simulink model "modelo_real"  (R2018b)
settings: Solver=ode4  StartTime=0.0  StopTime=t_f  FixedStep=fst  RelTol=1e-3
values from neighbouring files (symbols this model uses):
  b = 0.1210    (= 0.121)    [script_principal.m]
  c_d = r_d/(2*b)    (= 0.120661157025)    [script_principal.m]
  c_e = r_e/(2*b)    (= 0.121074380165)    [script_principal.m]
  delayD = 0.1/fst    (= 100)    [script_principal.m]
  delayE = 0.1/fst    (= 100)    [script_principal.m]
  filter_order = 2    [script_principal.m]
  freq_pos = 200    [script_principal.m]
  freq_vel = 200    [script_principal.m]
  k0 = 10    [script_principal.m]
  k_enc = 2*pi/fpr    (= 0.157079632679)    [script_principal.m]
  KaD_v = var_KaD*0.4713    (= 0.4713)    [script_principal.m]
  KaE_v = var_KaE*0.5046    (= 0.5046)    [script_principal.m]
  L = 0.1    [script_principal.m]
  svzD = 0    [script_principal.m]
  svzE = 0    [script_principal.m]
  T = 3    [script_principal.m]
  VaD_max = 14    [script_principal.m]
  VaD_min = 2    [script_principal.m]
  VaE_max = 14    [script_principal.m]
  VaE_min = 2    [script_principal.m]
  x0_1 = 0    [script_principal.m]
  x0_2 = 0    [script_principal.m]
  x0_3 = 0    [script_principal.m]
undefined symbols (not defined in the file or in its folder): a, dur_c, t_f, t_i, t_i_1, t_i_2, t_i_3, t_i_c, time_c, v, w, wx, wy
libraries: simulink x39, embdlinuxlib x7, cstblocks x4, dspmtrx3 x2, raspberrypilib x1
settings Model: SimulationMode=external  ExtModeTrigDuration=2  Creator=nenem  LastModifiedBy=nenem
settings SolverCC: PositivePriorityOrder=on
settings OptimizationCC: EnhancedBackFolding=on  PassReuseOutputArgsAs=Individual arguments  MaxStackSize=64  OptimizeBlockOrder=speed  DifferentSizesBufferReuse=on  OptimizationCustomize=off
settings DebuggingCC: ParameterTunabilityLossMsg=error
settings HardwareCC: ProdBitPerPointer=32  ProdBitPerSizeT=32  ProdBitPerPtrDiffT=32  ProdLargestAtomicInteger=Long  ProdLargestAtomicFloat=Double  ProdWordSize=32  ProdHWDeviceType=ARM Compatible->ARM Cortex
settings SFSimCC: MATLABDynamicMemAlloc=off
settings RTWCC: SystemTargetFile=ert.tlc  HardwareBoard=Raspberry Pi  TLCOptions="-aInlineSetEventsForThisBaseRateFcn=TLC_FALSE -aSuppressMultiTaskScheduler=TLC_FALSE  -aRateBasedStepFcn=0"  TemplateMakefile=ert_default_tmf  GenerateReport=on  Toolchain=GNU GCC Raspberry Pi  BuildConfiguration=Faster Runs  IncludeHyperlinkInReport=on  LaunchReport=on  GenerateTraceInfo=on  GenerateTraceReport=on  GenerateTraceReportSl=on  GenerateTraceReportSf=on  GenerateTraceReportEml=on
settings CodeAppCC: ForceParamTrailComments=on  IgnoreCustomStorageClasses=off  OperatorAnnotations=on  SimulinkDataObjDesc=on  SFDataObjDesc=on  InsertBlockDesc=on
settings ERTTargetCC: SupportContinuousTime=on  SupportVariableSizeSignals=on

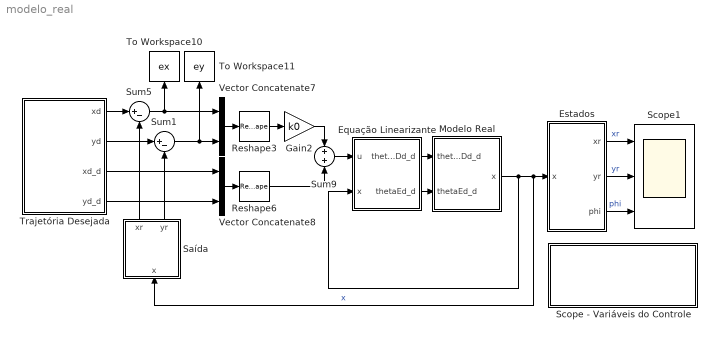
== system modelo_real ==
  Equação Linearizante : Subsystem
  Estados : Subsystem
  Gain2 : Gain  Gain=k0
  Modelo Real : Subsystem
  Reshape3 : Reshape  OutputDimensionality=Customize  OutputDimensions=[2,1]
  Reshape6 : Reshape  OutputDimensionality=Customize  OutputDimensions=[2,1]
  Saída : Subsystem
  Scope - Variáveis do Controle : Subsystem
  Scope1 : Scope  NumInputPorts=3
  Sum1 : Sum  Inputs=|+-
  Sum5 : Sum  Inputs=|+-
  Sum9 : Sum  Inputs=+|+
  To Workspace10 : ToWorkspace  VariableName=ex  SaveFormat=Structure With Time  SampleTime=-1
      settings: Save2DSignal=2-D array (concatenate along first dimension)
  To Workspace11 : ToWorkspace  VariableName=ey  SaveFormat=Structure With Time  SampleTime=-1
      settings: Save2DSignal=2-D array (concatenate along first dimension)
  Trajetória Desejada : Subsystem
  Vector Concatenate7 : Concatenate
  Vector Concatenate8 : Concatenate
  wires:
  Trajetória Desejada/1(xd) -> Sum5/1
  Sum1/1 -> To Workspace11/1, Vector Concatenate7/2
  Gain2/1 -> Sum9/1
  Reshape6/1 -> Sum9/2
  Estados/2(yr) -> Scope1/2  "yr"
  Sum5/1 -> To Workspace10/1, Vector Concatenate7/1
  Trajetória Desejada/4(yd_d) -> Vector Concatenate8/2
  Trajetória Desejada/3(xd_d) -> Vector Concatenate8/1
  Trajetória Desejada/2(yd) -> Sum1/1
  Vector Concatenate7/1 -> Reshape3/1
  Estados/1(xr) -> Scope1/1  "xr"
  Reshape3/1 -> Gain2/1
  Sum9/1 -> Equação Linearizante/1(u)
  Saída/2(yr) -> Sum1/2
  Vector Concatenate8/1 -> Reshape6/1
  Modelo Real/1(x) -> Equação Linearizante/2(x), Saída/1(x), Estados/1(x)  "x"
  Saída/1(xr) -> Sum5/2
  Estados/3(phi) -> Scope1/3  "phi"
  Equação Linearizante/2(thetaEd_d) -> Modelo Real/2(thetaEd_d)
  Equação Linearizante/1(thetaDd_d) -> Modelo Real/1(thetaDd_d)

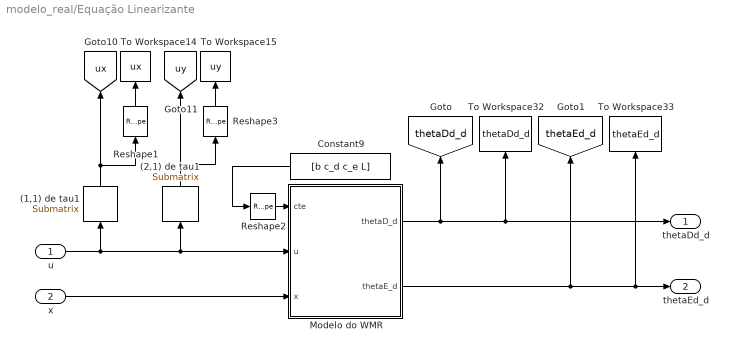
== system modelo_real/Equação Linearizante ==
  u : Inport
  x : Inport  Port=2
  (1,1) de tau1 : dspmtrx3/Submatrix  RowSpan=One row  RowStartMode=Index  RowStartIndex=1  RowEndMode=Last  RowEndIndex=1  ColSpan=One column  ColStartMode=Index  ColStartIndex=1  ColEndMode=Last  ColEndIndex=1
  (2,1) de tau1 : dspmtrx3/Submatrix  RowSpan=One row  RowStartMode=Index  RowStartIndex=2  RowEndMode=Last  RowEndIndex=1  ColSpan=One column  ColStartMode=Index  ColStartIndex=1  ColEndMode=Last  ColEndIndex=1
  Constant9 : Constant  Value=[b c_d c_e L]
  Modelo do WMR : MATLAB Function  TreatAsAtomicUnit=on
  Reshape1 : Reshape
  Reshape2 : Reshape  OutputDimensionality=Customize  OutputDimensions=[1,4]
  Reshape3 : Reshape
  To Workspace14 : ToWorkspace  VariableName=ux  SaveFormat=Structure With Time  SampleTime=-1
      settings: Save2DSignal=2-D array (concatenate along first dimension)
  To Workspace15 : ToWorkspace  VariableName=uy  SaveFormat=Structure With Time  SampleTime=-1
      settings: Save2DSignal=2-D array (concatenate along first dimension)
  To Workspace32 : ToWorkspace  VariableName=thetaDd_d  SaveFormat=Structure With Time  SampleTime=-1
      settings: Save2DSignal=2-D array (concatenate along first dimension)
  To Workspace33 : ToWorkspace  VariableName=thetaEd_d  SaveFormat=Structure With Time  SampleTime=-1
      settings: Save2DSignal=2-D array (concatenate along first dimension)
  thetaDd_d : Outport
  thetaEd_d : Outport  Port=2
  tag scope: thetaDd_d=global, thetaEd_d=global, ux=global, uy=global
  wires:
  x/1 -> Modelo do WMR/3(x)
  Reshape2/1 -> Modelo do WMR/1(cte)
  Constant9/1 -> Reshape2/1
  u/1 -> (1,1) de tau1/1, (2,1) de tau1/1, Modelo do WMR/2(u)
  (2,1) de tau1/1 -> Reshape3/1, [uy]
  (1,1) de tau1/1 -> Reshape1/1, [ux]
  Modelo do WMR/1(thetaD_d) -> [thetaDd_d], To Workspace32/1, thetaDd_d/1
  Modelo do WMR/2(thetaE_d) -> thetaEd_d/1, To Workspace33/1, [thetaEd_d]
  Reshape1/1 -> To Workspace14/1
  Reshape3/1 -> To Workspace15/1

== system modelo_real/Estados ==
  x : Inport
  Estados : MATLAB Function  TreatAsAtomicUnit=on
  To Workspace2 : ToWorkspace  VariableName=phi  SaveFormat=Structure With Time  SampleTime=-1
      settings: Save2DSignal=2-D array (concatenate along first dimension)
  To Workspace3 : ToWorkspace  VariableName=xr  SaveFormat=Structure With Time  SampleTime=-1
      settings: Save2DSignal=2-D array (concatenate along first dimension)
  To Workspace4 : ToWorkspace  VariableName=yr  SaveFormat=Structure With Time  SampleTime=-1
      settings: Save2DSignal=2-D array (concatenate along first dimension)
  xr : Outport
  yr : Outport  Port=2
  phi : Outport  Port=3
  tag scope: phi=global, xr=global, yr=global
  wires:
  x/1 -> Estados/1(x)
  Estados/1(xr) -> xr/1, To Workspace3/1, [xr]
  Estados/2(yr) -> [yr], yr/1, To Workspace4/1
  Estados/3(phi) -> phi/1, To Workspace2/1, [phi]

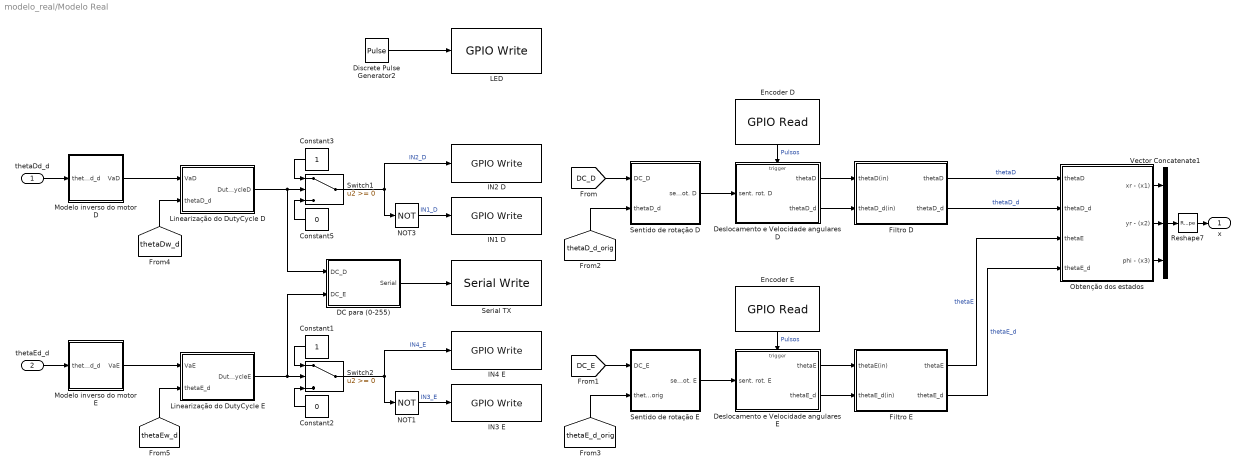
== system modelo_real/Modelo Real ==
  thetaDd_d : Inport
  thetaEd_d : Inport  Port=2
  Constant1 : Constant
  Constant2 : Constant  Value=0
  Constant3 : Constant
  Constant5 : Constant  Value=0
  DC para (0-255) : Subsystem
  Deslocamento e Velocidade angulares D : Subsystem  TreatAsAtomicUnit=on
  Deslocamento e Velocidade angulares E : Subsystem  TreatAsAtomicUnit=on
  Discrete Pulse Generator2 : DiscretePulseGenerator  SampleTime=0.25
  Encoder D : embdlinuxlib/GPIO Read  board=Pi 3 Model B  gpio=26  internalResistor=Off  sampleTime=0.001  direction=Input  blockPlatform=Raspberry Pi
      settings: SourceProductName=Simulink Support Package for Raspberry Pi Hardware  SourceProductBaseCode=RASPPI
  Encoder E : embdlinuxlib/GPIO Read  board=Pi 3 Model B  gpio=5  internalResistor=Off  sampleTime=0.001  direction=Input  blockPlatform=Raspberry Pi
      settings: SourceProductName=Simulink Support Package for Raspberry Pi Hardware  SourceProductBaseCode=RASPPI
  Filtro D : Subsystem
  Filtro E : Subsystem
  IN1 D : embdlinuxlib/GPIO Write  board=Pi 3 Model B  gpio=16  direction=Output  blockPlatform=Raspberry Pi
      settings: SourceProductName=Simulink Support Package for Raspberry Pi Hardware  SourceProductBaseCode=RASPPI
  IN2 D : embdlinuxlib/GPIO Write  board=Pi 3 Model B  gpio=20  direction=Output  blockPlatform=Raspberry Pi
      settings: SourceProductName=Simulink Support Package for Raspberry Pi Hardware  SourceProductBaseCode=RASPPI
  IN3 E : embdlinuxlib/GPIO Write  board=Pi 3 Model B  gpio=19  direction=Output  blockPlatform=Raspberry Pi
      settings: SourceProductName=Simulink Support Package for Raspberry Pi Hardware  SourceProductBaseCode=RASPPI
  IN4 E : embdlinuxlib/GPIO Write  board=Pi 3 Model B  gpio=6  direction=Output  blockPlatform=Raspberry Pi
      settings: SourceProductName=Simulink Support Package for Raspberry Pi Hardware  SourceProductBaseCode=RASPPI
  LED : embdlinuxlib/GPIO Write  board=Pi 3 Model B  gpio=21  direction=Output  blockPlatform=Raspberry Pi
      settings: SourceProductName=Simulink Support Package for Raspberry Pi Hardware  SourceProductBaseCode=RASPPI
  Linearização do DutyCycle D : Subsystem
  Linearização do DutyCycle E : Subsystem
  Modelo inverso do motor D : Subsystem
  Modelo inverso do motor E : Subsystem
  NOT1 : Logic  Operator=NOT  IconShape=distinctive  AllPortsSameDT=off  OutDataTypeStr=boolean
  NOT3 : Logic  Operator=NOT  IconShape=distinctive  AllPortsSameDT=off  OutDataTypeStr=boolean
  Obtenção dos estados : Subsystem
  Reshape7 : Reshape  OutputDimensionality=Customize  OutputDimensions=[3,1]
  Sentido de rotação D : Subsystem
  Sentido de rotação E : Subsystem
  Serial TX : raspberrypilib/Serial Write  board=Pi 3 Model B  SCIModule_=/dev/ttyS0  Baudrate_=230400  Parity=None  StopBits_=1  HardwareFlowControl=None  ByteOrder=LittleEndian  OutputStatus=off  blockPlatform=RaspberryPi
      settings: SourceProductName=Simulink Support Package for Raspberry Pi Hardware  SourceProductBaseCode=RASPPI
  Switch1 : Switch
  Switch2 : Switch
  Vector Concatenate1 : Concatenate  NumInputs=3
  x : Outport
  wires:
  Filtro D/1(thetaD) -> Obtenção dos estados/1(thetaD)  "thetaD"
  Switch1/1 -> IN2 D/1, NOT3/1  "IN2_D"
  Filtro E/1(thetaE) -> Obtenção dos estados/3(thetaE)  "thetaE"
  Sentido de rotação D/1(sent. rot. D) -> Deslocamento e Velocidade angulares D/1(sent. rot. D)
  Sentido de rotação E/1(sent. rot. E) -> Deslocamento e Velocidade angulares E/1(sent. rot. E)
  Encoder E/1 -> Deslocamento e Velocidade angulares E/Trigger  "Pulsos"
  NOT3/1 -> IN1 D/1  "IN1_D"
  Switch2/1 -> IN4 E/1, NOT1/1  "IN4_E"
  [DC_D] -> Sentido de rotação D/1(DC_D)
  Encoder D/1 -> Deslocamento e Velocidade angulares D/Trigger  "Pulsos"
  Discrete Pulse Generator2/1 -> LED/1
  Vector Concatenate1/1 -> Reshape7/1
  Filtro D/2(thetaD_d) -> Obtenção dos estados/2(thetaD_d)  "thetaD_d"
  Filtro E/2(thetaE_d) -> Obtenção dos estados/4(thetaE_d)  "thetaE_d"
  [DC_E] -> Sentido de rotação E/1(DC_E)
  thetaDd_d/1 -> Modelo inverso do motor D/1(thetaDd_d)
  Modelo inverso do motor D/1(VaD) -> Linearização do DutyCycle D/1(VaD)
  Linearização do DutyCycle D/1(DutyCycleD) -> DC para (0-255)/1(DC_D), Switch1/2
  thetaEd_d/1 -> Modelo inverso do motor E/1(thetaEd_d)
  Modelo inverso do motor E/1(VaE) -> Linearização do DutyCycle E/1(VaE)
  Linearização do DutyCycle E/1(DutyCycleE) -> DC para (0-255)/2(DC_E), Switch2/2
  DC para (0-255)/1(Serial) -> Serial TX/1
  Constant3/1 -> Switch1/1
  Constant5/1 -> Switch1/3
  Constant1/1 -> Switch2/1
  Constant2/1 -> Switch2/3
  Deslocamento e Velocidade angulares D/1(thetaD) -> Filtro D/1(thetaD(in))
  Deslocamento e Velocidade angulares D/2(thetaD_d) -> Filtro D/2(thetaD_d(in))
  Deslocamento e Velocidade angulares E/1(thetaE) -> Filtro E/1(thetaE(in))
  Deslocamento e Velocidade angulares E/2(thetaE_d) -> Filtro E/2(thetaE_d(in))
  Reshape7/1 -> x/1
  Obtenção dos estados/1(xr - (x1)) -> Vector Concatenate1/1
  Obtenção dos estados/2(yr - (x2)) -> Vector Concatenate1/2
  Obtenção dos estados/3(phi - (x3)) -> Vector Concatenate1/3
  NOT1/1 -> IN3 E/1  "IN3_E"
  [thetaD_d_orig] -> Sentido de rotação D/2(thetaD_d)
  [thetaE_d_orig] -> Sentido de rotação E/2(thetaE_d_orig)
  [thetaDw_d] -> Linearização do DutyCycle D/2(thetaD_d)
  [thetaEw_d] -> Linearização do DutyCycle E/2(thetaE_d)

== system modelo_real/Saída ==
  x : Inport
  Reshape1 : Reshape  OutputDimensionality=Customize  OutputDimensions=[3,1]
  Saídas : MATLAB Function  TreatAsAtomicUnit=on
  xr : Outport
  yr : Outport  Port=2
  wires:
  x/1 -> Reshape1/1
  Saídas/1(xr) -> xr/1
  Saídas/2(yr) -> yr/1
  Reshape1/1 -> Saídas/1(x)

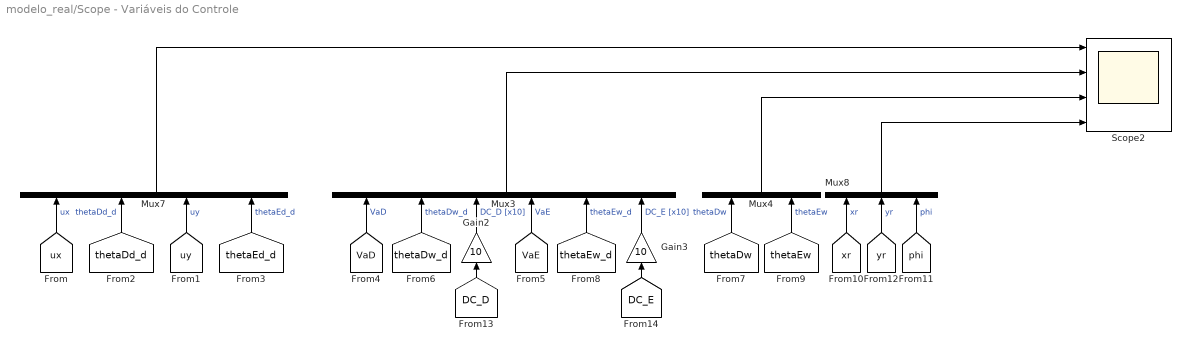
== system modelo_real/Scope - Variáveis do Controle ==
  Gain2 : Gain  Gain=10
  Gain3 : Gain  Gain=10
  Mux3 : Mux  Inputs=6
  Mux4 : Mux  Inputs=2
  Mux7 : Mux
  Mux8 : Mux  Inputs=3
  Scope2 : Scope  NumInputPorts=4
  wires:
  [ux] -> Mux7/1  "ux"
  [thetaDw] -> Mux4/1  "thetaDw"
  [thetaEw_d] -> Mux3/5  "thetaEw_d"
  [phi] -> Mux8/3  "phi"
  [thetaDw_d] -> Mux3/2  "thetaDw_d"
  Mux4/1 -> Scope2/3
  [xr] -> Mux8/1  "xr"
  [thetaEw] -> Mux4/2  "thetaEw"
  Mux7/1 -> Scope2/1
  [yr] -> Mux8/2  "yr"
  [uy] -> Mux7/3  "uy"
  [thetaEd_d] -> Mux7/4  "thetaEd_d"
  Mux8/1 -> Scope2/4
  [VaE] -> Mux3/4  "VaE"
  [VaD] -> Mux3/1  "VaD"
  [thetaDd_d] -> Mux7/2  "thetaDd_d"
  Mux3/1 -> Scope2/2
  [DC_D] -> Gain2/1
  [DC_E] -> Gain3/1
  Gain2/1 -> Mux3/3  "DC_D [x10]"
  Gain3/1 -> Mux3/6  "DC_E [x10]"

== system modelo_real/Trajetória Desejada ==
  Hypot : Math  Operator=hypot  OutputSignalType=real  SaturateOnIntegerOverflow=on
  Integrator : Integrator
  Integrator1 : Integrator
  To Workspace : ToWorkspace  VariableName=vd  SaveFormat=Structure With Time  SampleTime=-1
      settings: Save2DSignal=2-D array (concatenate along first dimension)
  To Workspace1 : ToWorkspace  VariableName=xd  SaveFormat=Structure With Time  SampleTime=-1
      settings: Save2DSignal=2-D array (concatenate along first dimension)
  To Workspace2 : ToWorkspace  VariableName=yd  SaveFormat=Structure With Time  SampleTime=-1
      settings: Save2DSignal=2-D array (concatenate along first dimension)
  To Workspace5 : ToWorkspace  VariableName=xd_d  SaveFormat=Structure With Time  SampleTime=-1
      settings: Save2DSignal=2-D array (concatenate along first dimension)
  To Workspace6 : ToWorkspace  VariableName=yd_d  SaveFormat=Structure With Time  SampleTime=-1
      settings: Save2DSignal=2-D array (concatenate along first dimension)
  Velocidade da trajetória : Subsystem
  xd : Outport
  yd : Outport  Port=2
  xd_d : Outport  Port=3
  yd_d : Outport  Port=4
  wires:
  Integrator/1 -> xd/1, To Workspace1/1  "xd"
  Integrator1/1 -> yd/1, To Workspace2/1  "yd"
  Hypot/1 -> To Workspace/1
  Velocidade da trajetória/1(xd_d) -> Integrator/1, xd_d/1, To Workspace5/1, Hypot/1  "xd_d"
  Velocidade da trajetória/2(yd_d) -> Integrator1/1, yd_d/1, To Workspace6/1, Hypot/2  "yd_d"

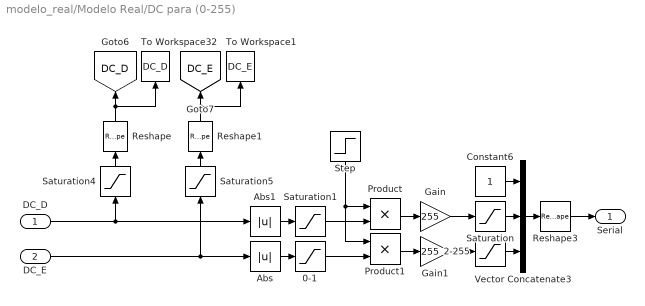
== system modelo_real/Modelo Real/DC para (0-255) ==
  DC_D : Inport
  DC_E : Inport  Port=2
  0-1 : Saturate  UpperLimit=1  LowerLimit=0
  2-255 : Saturate  UpperLimit=255  LowerLimit=2
  Abs : Abs
  Abs1 : Abs
  Constant6 : Constant  OutDataTypeStr=uint8
  Gain : Gain  Gain=255  OutDataTypeStr=uint8
  Gain1 : Gain  Gain=255  OutDataTypeStr=uint8
  Product : Product
  Product1 : Product
  Reshape : Reshape
  Reshape1 : Reshape
  Reshape3 : Reshape  OutputDimensionality=Column vector (2-D)  OutputDimensions=[3,1]
  Saturation : Saturate  UpperLimit=255  LowerLimit=2
  Saturation1 : Saturate  UpperLimit=1  LowerLimit=0
  Saturation4 : Saturate  UpperLimit=1  LowerLimit=-1
  Saturation5 : Saturate  UpperLimit=1  LowerLimit=-1
  Step : Step  Time=t_f-0.01  Before=1  After=0  SampleTime=0
  To Workspace1 : ToWorkspace  VariableName=DC_E  SaveFormat=Structure With Time  SampleTime=-1
      settings: Save2DSignal=2-D array (concatenate along first dimension)
  To Workspace32 : ToWorkspace  VariableName=DC_D  SaveFormat=Structure With Time  SampleTime=-1
      settings: Save2DSignal=2-D array (concatenate along first dimension)
  Vector Concatenate3 : Concatenate  NumInputs=3  ConcatenateDimension=5
  Serial : Outport
  tag scope: DC_D=global, DC_E=global
  wires:
  DC_E/1 -> Abs/1, Saturation5/1
  Saturation/1 -> Vector Concatenate3/2
  DC_D/1 -> Abs1/1, Saturation4/1
  Constant6/1 -> Vector Concatenate3/1
  2-255/1 -> Vector Concatenate3/3
  Vector Concatenate3/1 -> Reshape3/1
  Reshape3/1 -> Serial/1
  Saturation4/1 -> Reshape/1
  Saturation5/1 -> Reshape1/1
  Abs/1 -> 0-1/1
  Abs1/1 -> Saturation1/1
  0-1/1 -> Product1/2
  Saturation1/1 -> Product/2
  Reshape/1 -> To Workspace32/1, [DC_D]
  Reshape1/1 -> To Workspace1/1, [DC_E]
  Gain/1 -> Saturation/1
  Gain1/1 -> 2-255/1
  Step/1 -> Product1/1, Product/1
  Product/1 -> Gain/1
  Product1/1 -> Gain1/1

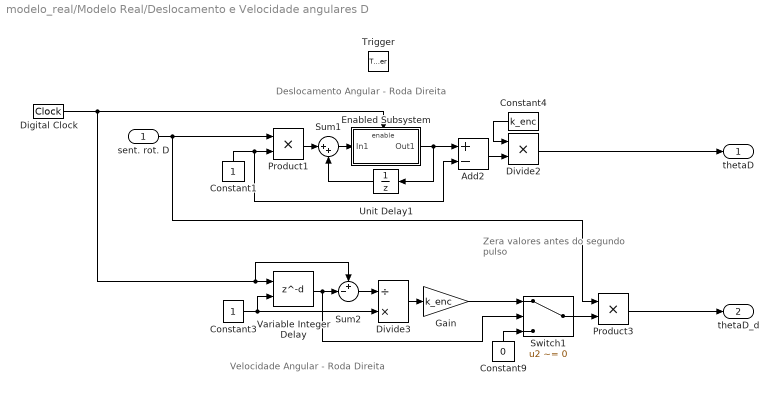
== system modelo_real/Modelo Real/Deslocamento e Velocidade angulares D ==
  note: Deslocamento Angular - Roda Direita
  note: Velocidade Angular - Roda Direita
  note: Zera valores antes
      | do segundo pulso
  sent. rot. D : Inport  LatchByDelayingOutsideSignal=on
  Trigger : TriggerPort  VariantControl=Variant
  Add2 : Sum  Inputs=+-
  Constant1 : Constant  OutDataTypeStr=double
  Constant3 : Constant  OutDataTypeStr=double
  Constant4 : Constant  Value=k_enc  OutDataTypeStr=double
  Constant9 : Constant  Value=0  OutDataTypeStr=double
  Digital Clock : DigitalClock  SampleTime=-1
  Divide2 : Product  Inputs=**  RndMeth=Nearest
  Divide3 : Product  Inputs=/*  RndMeth=Nearest
  Enabled Subsystem : Subsystem  TreatAsAtomicUnit=on
  Gain : Gain  Gain=k_enc
  Product1 : Product
  Product3 : Product
  Sum1 : Sum  Inputs=|++
  Sum2 : Sum  Inputs=+-|
  Switch1 : Switch  Criteria=u2 ~= 0
  Unit Delay1 : UnitDelay  SampleTime=-1
  Variable Integer Delay : Delay  DelayLengthSource=Input port
      settings: InputPortMap=u0,p1
  thetaD : Outport
  thetaD_d : Outport  Port=2
  wires:
  Constant1/1 -> Add2/2, Product1/2
  Enabled Subsystem/1(Out1) -> Add2/1, Unit Delay1/1
  Sum1/1 -> Enabled Subsystem/1(In1)
  Add2/1 -> Divide2/2
  Unit Delay1/1 -> Sum1/2
  Constant4/1 -> Divide2/1
  Product1/1 -> Sum1/1
  Divide3/1 -> Gain/1
  Digital Clock/1 -> Enabled Subsystem/Enable, Variable Integer Delay/1, Sum2/1
  Constant9/1 -> Switch1/3
  Variable Integer Delay/1 -> Sum2/2, Switch1/2
  Switch1/1 -> Product3/2
  Sum2/1 -> Divide3/1
  sent. rot. D/1 -> Product1/1, Product3/1
  Gain/1 -> Switch1/1
  Product3/1 -> thetaD_d/1
  Constant3/1 -> Divide3/2, Variable Integer Delay/2
  Divide2/1 -> thetaD/1

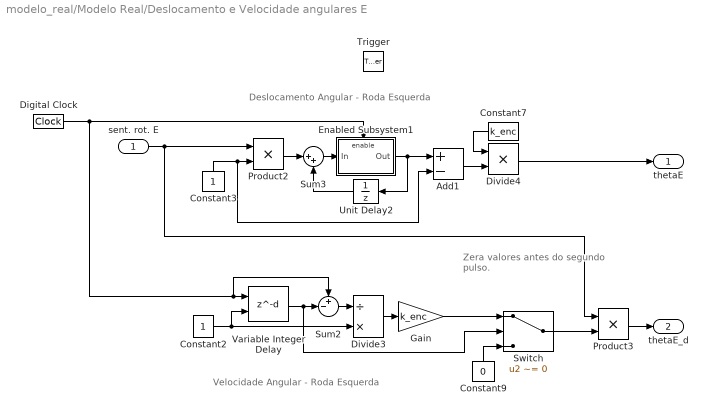
== system modelo_real/Modelo Real/Deslocamento e Velocidade angulares E ==
  note: Deslocamento Angular - Roda Esquerda
  note: Zera valores antes
      | do segundo pulso.
  note: Velocidade Angular - Roda Esquerda
  sent. rot. E : Inport  LatchByDelayingOutsideSignal=on
  Trigger : TriggerPort  VariantControl=Variant
  Add1 : Sum  Inputs=+-
  Constant2 : Constant  OutDataTypeStr=double
  Constant3 : Constant  OutDataTypeStr=double
  Constant7 : Constant  Value=k_enc  OutDataTypeStr=double
  Constant9 : Constant  Value=0  OutDataTypeStr=double
  Digital Clock : DigitalClock  SampleTime=-1
  Divide3 : Product  Inputs=/*  RndMeth=Nearest
  Divide4 : Product  Inputs=**  RndMeth=Nearest
  Enabled Subsystem1 : Subsystem  TreatAsAtomicUnit=on
  Gain : Gain  Gain=k_enc
  Product2 : Product
  Product3 : Product
  Sum2 : Sum  Inputs=+-|
  Sum3 : Sum  Inputs=|++
  Switch : Switch  Criteria=u2 ~= 0
  Unit Delay2 : UnitDelay  SampleTime=-1
  Variable Integer Delay : Delay  DelayLengthSource=Input port
      settings: InputPortMap=u0,p1
  thetaE : Outport
  thetaE_d : Outport  Port=2
  wires:
  Constant2/1 -> Divide3/2, Variable Integer Delay/2
  Product2/1 -> Sum3/1
  Digital Clock/1 -> Enabled Subsystem1/Enable, Variable Integer Delay/1, Sum2/1
  Sum2/1 -> Divide3/1
  Add1/1 -> Divide4/2
  Constant7/1 -> Divide4/1
  Sum3/1 -> Enabled Subsystem1/1(In)
  Constant9/1 -> Switch/3
  Enabled Subsystem1/1(Out) -> Add1/1, Unit Delay2/1
  Switch/1 -> Product3/2
  Unit Delay2/1 -> Sum3/2
  Variable Integer Delay/1 -> Switch/2, Sum2/2
  Constant3/1 -> Add1/2, Product2/2
  sent. rot. E/1 -> Product3/1, Product2/1
  Divide3/1 -> Gain/1
  Gain/1 -> Switch/1
  Product3/1 -> thetaE_d/1
  Divide4/1 -> thetaE/1

== system modelo_real/Modelo Real/Filtro D ==
  thetaD(in) : Inport
  thetaD_d(in) : Inport  Port=2
  Constant : Constant  Value=freq_vel
  Constant1 : Constant  Value=freq_pos
  Constant6 : Constant  Value=0
  Manual Switch : ManualSwitch  CurrentSetting=0
  Média : MATLAB Function  TreatAsAtomicUnit=on
  Sum : Sum  Inputs=+-|
  Switch3 : Switch  Criteria=u2 ~= 0
  Tapped Delay : simulink/Discrete/Tapped Delay  vinit=0.0  samptime=fst  NumDelays=delayD  DelayOrder=Oldest  includeCurrent=off
  To Workspace1 : ToWorkspace  VariableName=thetaD_orig  SaveFormat=Structure With Time  SampleTime=-1
      settings: Save2DSignal=2-D array (concatenate along first dimension)
  To Workspace32 : ToWorkspace  VariableName=thetaD_d_orig  SaveFormat=Structure With Time  SampleTime=-1
      settings: Save2DSignal=2-D array (concatenate along first dimension)
  Unit Delay2 : UnitDelay  SampleTime=-1
  Varying Lowpass Filter : cstblocks/Linear Parameter Varying/Varying Lowpass Filter  N=filter_order
      settings: SourceProductName=Control System Toolbox
  Varying Lowpass Filter1 : cstblocks/Linear Parameter Varying/Varying Lowpass Filter  N=filter_order
      settings: SourceProductName=Control System Toolbox
  thetaD : Outport
  thetaD_d : Outport  Port=2
  tag scope: thetaD_d_orig=global
  wires:
  Constant6/1 -> Switch3/3
  Média/1(y) -> Sum/1, Unit Delay2/1
  thetaD_d(in)/1 -> Switch3/1
  Tapped Delay/1 -> Média/1(u)
  Unit Delay2/1 -> Sum/2
  Sum/1 -> Switch3/2  "Δpos"
  Constant/1 -> Varying Lowpass Filter/2
  Switch3/1 -> Varying Lowpass Filter/1, [thetaD_d_orig], To Workspace32/1
  Varying Lowpass Filter/1 -> thetaD_d/1
  Constant1/1 -> Varying Lowpass Filter1/2
  thetaD(in)/1 -> Manual Switch/1, Varying Lowpass Filter1/1, To Workspace1/1, Tapped Delay/1
  Manual Switch/1 -> thetaD/1
  Varying Lowpass Filter1/1 -> Manual Switch/2

== system modelo_real/Modelo Real/Filtro E ==
  thetaE(in) : Inport
  thetaE_d(in) : Inport  Port=2
  Constant : Constant  Value=freq_vel
  Constant1 : Constant  Value=freq_pos
  Constant6 : Constant  Value=0
  Manual Switch : ManualSwitch  CurrentSetting=0
  Média : MATLAB Function  TreatAsAtomicUnit=on
  Sum : Sum  Inputs=+-|
  Switch3 : Switch  Criteria=u2 ~= 0
  Tapped Delay : simulink/Discrete/Tapped Delay  vinit=0.0  samptime=fst  NumDelays=delayE  DelayOrder=Oldest  includeCurrent=off
  To Workspace1 : ToWorkspace  VariableName=thetaE_orig  SaveFormat=Structure With Time  SampleTime=-1
      settings: Save2DSignal=2-D array (concatenate along first dimension)
  To Workspace33 : ToWorkspace  VariableName=thetaE_d_orig  SaveFormat=Structure With Time  SampleTime=-1
      settings: Save2DSignal=2-D array (concatenate along first dimension)
  Unit Delay2 : UnitDelay  SampleTime=-1
  Varying Lowpass Filter : cstblocks/Linear Parameter Varying/Varying Lowpass Filter  N=filter_order
      settings: SourceProductName=Control System Toolbox
  Varying Lowpass Filter1 : cstblocks/Linear Parameter Varying/Varying Lowpass Filter  N=filter_order
      settings: SourceProductName=Control System Toolbox
  thetaE : Outport
  thetaE_d : Outport  Port=2
  tag scope: thetaE_d_orig=global
  wires:
  Constant6/1 -> Switch3/3
  Média/1(y) -> Sum/1, Unit Delay2/1
  thetaE_d(in)/1 -> Switch3/1
  Tapped Delay/1 -> Média/1(u)
  Unit Delay2/1 -> Sum/2
  Sum/1 -> Switch3/2  "Δpos"
  Constant/1 -> Varying Lowpass Filter/2
  Switch3/1 -> Varying Lowpass Filter/1, [thetaE_d_orig], To Workspace33/1
  Varying Lowpass Filter/1 -> thetaE_d/1
  Constant1/1 -> Varying Lowpass Filter1/2
  thetaE(in)/1 -> To Workspace1/1, Manual Switch/1, Varying Lowpass Filter1/1, Tapped Delay/1
  Manual Switch/1 -> thetaE/1
  Varying Lowpass Filter1/1 -> Manual Switch/2

== system modelo_real/Modelo Real/Linearização do DutyCycle D ==
  VaD : Inport
  thetaD_d : Inport  Port=2
  Abs : Abs
  Constant : Constant  Value=VaD_max
  Constant3 : Constant
  Constant5 : Constant  Value=-1
  Divide1 : Product  Inputs=*/
  Gain1 : Gain  Gain=KaD_v
  Product : Product
  Sum1 : Sum  Inputs=|+-
  Sum2 : Sum  Inputs=|+-
  Switch1 : Switch
  DutyCycleD : Outport
  wires:
  Sum2/1 -> Abs/1
  Constant5/1 -> Switch1/3
  Product/1 -> Sum2/1
  Sum1/1 -> Divide1/1
  thetaD_d/1 -> Gain1/1
  Constant/1 -> Product/1
  VaD/1 -> Switch1/2, Sum1/1
  Divide1/1 -> DutyCycleD/1
  Switch1/1 -> Product/2
  Constant3/1 -> Switch1/1
  Gain1/1 -> Sum1/2, Sum2/2  "f.c.e.m."
  Abs/1 -> Divide1/2

== system modelo_real/Modelo Real/Linearização do DutyCycle E ==
  VaE : Inport
  thetaE_d : Inport  Port=2
  Abs : Abs
  Constant1 : Constant  Value=-1
  Constant3 : Constant
  Constant5 : Constant  Value=VaE_max
  Divide : Product  Inputs=*/
  Gain12 : Gain  Gain=KaE_v
  Product : Product
  Sum4 : Sum  Inputs=|+-
  Sum5 : Sum  Inputs=|+-
  Switch1 : Switch
  DutyCycleE : Outport
  wires:
  Sum5/1 -> Abs/1
  Constant1/1 -> Switch1/3
  Product/1 -> Sum5/1
  Sum4/1 -> Divide/1
  thetaE_d/1 -> Gain12/1
  Constant5/1 -> Product/1
  VaE/1 -> Switch1/2, Sum4/1
  Divide/1 -> DutyCycleE/1
  Switch1/1 -> Product/2
  Constant3/1 -> Switch1/1
  Gain12/1 -> Sum4/2, Sum5/2  "f.c.e.m."
  Abs/1 -> Divide/2

== system modelo_real/Modelo Real/Modelo inverso do motor D ==
  thetaDd_d : Inport
  Abs : Abs
  Constant : Constant  Value=VaD_min
  Gain4 : Gain  Gain=KaD_v
  Product : Product
  Reshape1 : Reshape
  Step : Step  Time=t_i  SampleTime=0
  Switch : Switch  Threshold=VaD_min
  To Workspace22 : ToWorkspace  VariableName=VaD  SaveFormat=Structure With Time  SampleTime=-1
      settings: Save2DSignal=2-D array (concatenate along first dimension)
  VaD : Outport
  tag scope: VaD=global
  wires:
  thetaDd_d/1 -> Gain4/1
  Gain4/1 -> Switch/1, Abs/1
  Product/1 -> Reshape1/1, VaD/1, [VaD]
  Switch/1 -> Product/2
  Constant/1 -> Switch/3
  Abs/1 -> Switch/2
  Step/1 -> Product/1
  Reshape1/1 -> To Workspace22/1

== system modelo_real/Modelo Real/Modelo inverso do motor E ==
  thetaEd_d : Inport
  Abs : Abs
  Constant : Constant  Value=VaE_min
  Gain7 : Gain  Gain=KaE_v
  Product : Product
  Reshape1 : Reshape
  Step : Step  Time=t_i  SampleTime=0
  Switch : Switch  Threshold=VaE_min
  To Workspace23 : ToWorkspace  VariableName=VaE  SaveFormat=Structure With Time  SampleTime=-1
      settings: Save2DSignal=2-D array (concatenate along first dimension)
  VaE : Outport
  tag scope: VaE=global
  wires:
  thetaEd_d/1 -> Gain7/1
  Product/1 -> Reshape1/1, VaE/1, [VaE]
  Constant/1 -> Switch/3
  Switch/1 -> Product/2
  Gain7/1 -> Switch/1, Abs/1
  Abs/1 -> Switch/2
  Step/1 -> Product/1
  Reshape1/1 -> To Workspace23/1

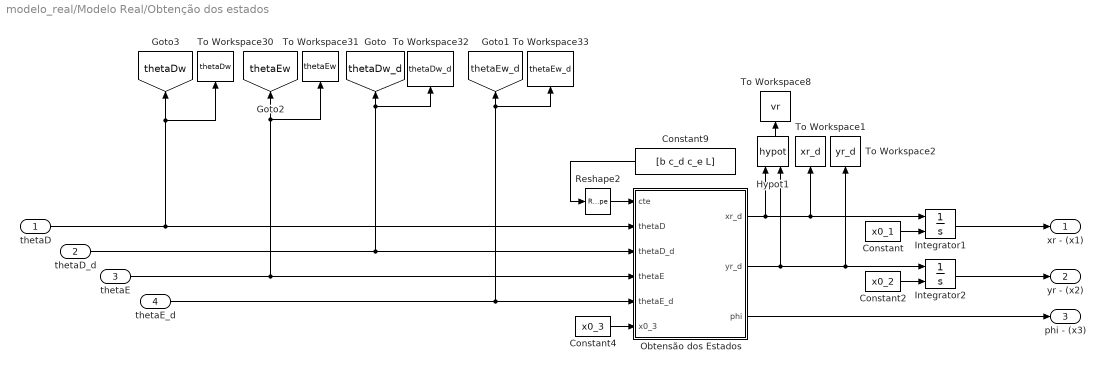
== system modelo_real/Modelo Real/Obtenção dos estados ==
  thetaD : Inport
  thetaD_d : Inport  Port=2
  thetaE : Inport  Port=3
  thetaE_d : Inport  Port=4
  Constant : Constant  Value=x0_1
  Constant2 : Constant  Value=x0_2
  Constant4 : Constant  Value=x0_3
  Constant9 : Constant  Value=[b c_d c_e L]
  Hypot1 : Math  Operator=hypot  SaturateOnIntegerOverflow=on
  Integrator1 : Integrator  InitialConditionSource=external
  Integrator2 : Integrator  InitialConditionSource=external
  Obtensão dos Estados : MATLAB Function  TreatAsAtomicUnit=on
  Reshape2 : Reshape  OutputDimensionality=Customize  OutputDimensions=[1,4]
  To Workspace1 : ToWorkspace  VariableName=xr_d  SaveFormat=Structure With Time  SampleTime=-1
      settings: Save2DSignal=2-D array (concatenate along first dimension)
  To Workspace2 : ToWorkspace  VariableName=yr_d  SaveFormat=Structure With Time  SampleTime=-1
      settings: Save2DSignal=2-D array (concatenate along first dimension)
  To Workspace30 : ToWorkspace  VariableName=thetaDw  SaveFormat=Structure With Time  SampleTime=-1
      settings: Save2DSignal=2-D array (concatenate along first dimension)
  To Workspace31 : ToWorkspace  VariableName=thetaEw  SaveFormat=Structure With Time  SampleTime=-1
      settings: Save2DSignal=2-D array (concatenate along first dimension)
  To Workspace32 : ToWorkspace  VariableName=thetaDw_d  SaveFormat=Structure With Time  SampleTime=-1
      settings: Save2DSignal=2-D array (concatenate along first dimension)
  To Workspace33 : ToWorkspace  VariableName=thetaEw_d  SaveFormat=Structure With Time  SampleTime=-1
      settings: Save2DSignal=2-D array (concatenate along first dimension)
  To Workspace8 : ToWorkspace  VariableName=vr  SaveFormat=Structure With Time  SampleTime=-1
      settings: Save2DSignal=2-D array (concatenate along first dimension)
  xr - (x1) : Outport
  yr - (x2) : Outport  Port=2
  phi - (x3) : Outport  Port=3
  tag scope: thetaDw=global, thetaDw_d=global, thetaEw=global, thetaEw_d=global
  wires:
  Obtensão dos Estados/1(xr_d) -> Hypot1/1, To Workspace1/1, Integrator1/1
  Integrator2/1 -> yr - (x2)/1
  Integrator1/1 -> xr - (x1)/1
  thetaE/1 -> Obtensão dos Estados/4(thetaE), [thetaEw], To Workspace31/1
  thetaE_d/1 -> Obtensão dos Estados/5(thetaE_d), To Workspace33/1, [thetaEw_d]
  thetaD_d/1 -> Obtensão dos Estados/3(thetaD_d), To Workspace32/1, [thetaDw_d]
  thetaD/1 -> Obtensão dos Estados/2(thetaD), To Workspace30/1, [thetaDw]
  Hypot1/1 -> To Workspace8/1
  Obtensão dos Estados/2(yr_d) -> Hypot1/2, To Workspace2/1, Integrator2/1
  Constant9/1 -> Reshape2/1
  Reshape2/1 -> Obtensão dos Estados/1(cte)
  Obtensão dos Estados/3(phi) -> phi - (x3)/1
  Constant2/1 -> Integrator2/2
  Constant/1 -> Integrator1/2
  Constant4/1 -> Obtensão dos Estados/6(x0_3)

== system modelo_real/Modelo Real/Sentido de rotação D ==
  DC_D : Inport
  thetaD_d : Inport  Port=2
  Abs : Abs
  Constant1 : Constant  Value=-1  OutDataTypeStr=double
  Constant4 : Constant  OutDataTypeStr=double
  Switch1 : Switch
  Switch2 : Switch  Criteria=u2 > Threshold  Threshold=svzD
  sent. rot. D : Outport
  wires:
  Switch1/1 -> sent. rot. D/1
  Switch2/1 -> Switch1/2
  Constant4/1 -> Switch1/1
  Constant1/1 -> Switch1/3
  Abs/1 -> Switch2/2
  DC_D/1 -> Switch2/3
  thetaD_d/1 -> Abs/1, Switch2/1

== system modelo_real/Modelo Real/Sentido de rotação E ==
  DC_E : Inport
  thetaE_d_orig : Inport  Port=2
  Abs : Abs
  Constant1 : Constant  Value=-1  OutDataTypeStr=double
  Constant4 : Constant  OutDataTypeStr=double
  Switch : Switch  Criteria=u2 > Threshold  Threshold=svzE
  Switch1 : Switch
  sent. rot. E : Outport
  wires:
  Switch1/1 -> sent. rot. E/1
  Switch/1 -> Switch1/2
  Constant4/1 -> Switch1/1
  Constant1/1 -> Switch1/3
  thetaE_d_orig/1 -> Abs/1, Switch/1
  Abs/1 -> Switch/2
  DC_E/1 -> Switch/3

== system modelo_real/Trajetória Desejada/Velocidade da trajetória ==
  0 : Subsystem  Commented=on
  0 c/ RAMPA : Subsystem  Commented=on
  180 c/ RAMPA : Subsystem
  8 : Subsystem  Commented=on
  "90 " : Subsystem  Commented=on
  90 c/ RAMPA : Subsystem  Commented=on
  Constant : Constant  Value=T
  Multiport Switch : MultiPortSwitch  Inputs=4
  Multiport Switch1 : MultiPortSwitch  Inputs=4
  Reta c/ RAMPA : Subsystem  Commented=on
  xd_d : Outport
  yd_d : Outport  Port=2
  wires:
  0 c/ RAMPA/2(yd_d) -> Multiport Switch1/2  "yd_d"
  90 c/ RAMPA/2(yd_d) -> Multiport Switch1/3  "yd_d"
  90 c/ RAMPA/1(xd_d) -> Multiport Switch/3  "xd_d"
  0 c/ RAMPA/1(xd_d) -> Multiport Switch/2  "xd_d"
  Constant/1 -> Multiport Switch/1, Multiport Switch1/1
  Multiport Switch/1 -> xd_d/1  "xd_d"
  Multiport Switch1/1 -> yd_d/1  "yd_d"
  8/2(yd_d) -> Multiport Switch1/5  "yd_d"
  180 c/ RAMPA/2(yd_d) -> Multiport Switch1/4  "yd_d"
  180 c/ RAMPA/1(xd_d) -> Multiport Switch/4  "xd_d"
  8/1(xd_d) -> Multiport Switch/5

== system modelo_real/Modelo Real/Deslocamento e Velocidade angulares D/Enabled Subsystem ==
  In1 : Inport
  Enable : EnablePort
  Out1 : Outport
  wires:
  In1/1 -> Out1/1

== system modelo_real/Modelo Real/Deslocamento e Velocidade angulares E/Enabled Subsystem1 ==
  In : Inport
  Enable : EnablePort
  Out : Outport
  wires:
  In/1 -> Out/1

== system modelo_real/Trajetória Desejada/Velocidade da trajetória/0 ==
  Gain : Gain  Gain=w
  Gain1 : Gain  Gain=v
  Gain2 : Gain  Gain=w
  Gain3 : Gain  Gain=v
  Gain4 : Gain  Gain=-1
  Ramp18 : simulink/Sources/Ramp  slope=1  start=t_i  InitialOutput=0
  Ramp19 : simulink/Sources/Ramp  slope=-1  start=t_i  InitialOutput=0
  Trigonometric Function : Trigonometry
  Trigonometric Function1 : Trigonometry  Operator=cos
  xd_d : Outport
  yd_d : Outport  Port=2
  wires:
  Gain4/1 -> Gain1/1
  Ramp18/1 -> Gain/1
  Gain/1 -> Trigonometric Function/1
  Trigonometric Function1/1 -> Gain3/1
  Gain2/1 -> Trigonometric Function1/1
  Ramp19/1 -> Gain2/1
  Gain1/1 -> xd_d/1
  Gain3/1 -> yd_d/1
  Trigonometric Function/1 -> Gain4/1

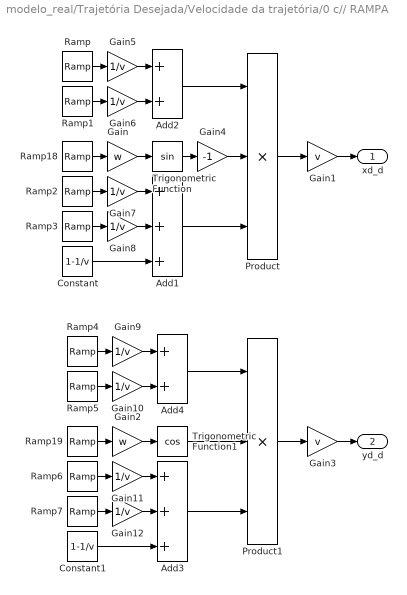
== system modelo_real/Trajetória Desejada/Velocidade da trajetória/0 c// RAMPA ==
  Add1 : Sum  Inputs=3
  Add2 : Sum  Inputs=2
  Add3 : Sum  Inputs=3
  Add4 : Sum  Inputs=2
  Constant : Constant  Value=1-1/v
  Constant1 : Constant  Value=1-1/v
  Gain : Gain  Gain=w
  Gain1 : Gain  Gain=v
  Gain{5..12} (8 alike) : Gain  Gain=1/v
  Gain2 : Gain  Gain=w
  Gain3 : Gain  Gain=v
  Gain4 : Gain  Gain=-1
  Product : Product  Inputs=3
  Product1 : Product  Inputs=3
  Ramp : simulink/Sources/Ramp  slope=a  start=t_i  InitialOutput=0
  Ramp1 : simulink/Sources/Ramp  slope=-a  start=t_1  InitialOutput=0
  Ramp18 : simulink/Sources/Ramp  slope=1  start=t_i  InitialOutput=0
  Ramp19 : simulink/Sources/Ramp  slope=1  start=t_i  InitialOutput=0
  Ramp2 : simulink/Sources/Ramp  slope=-a  start=t_2  InitialOutput=1
  Ramp3 : simulink/Sources/Ramp  slope=a  start=t_f  InitialOutput=0
  Ramp4 : simulink/Sources/Ramp  slope=a  start=t_i  InitialOutput=0
  Ramp5 : simulink/Sources/Ramp  slope=-a  start=t_1  InitialOutput=0
  Ramp6 : simulink/Sources/Ramp  slope=-a  start=t_2  InitialOutput=1
  Ramp7 : simulink/Sources/Ramp  slope=a  start=t_f  InitialOutput=0
  Trigonometric Function : Trigonometry
  Trigonometric Function1 : Trigonometry  Operator=cos
  xd_d : Outport
  yd_d : Outport  Port=2
  wires:
  Product/1 -> Gain1/1
  Ramp18/1 -> Gain/1
  Gain/1 -> Trigonometric Function/1
  Gain2/1 -> Trigonometric Function1/1
  Ramp19/1 -> Gain2/1
  Gain1/1 -> xd_d/1
  Gain3/1 -> yd_d/1
  Trigonometric Function/1 -> Gain4/1
  Ramp/1 -> Gain5/1
  Ramp1/1 -> Gain6/1
  Gain5/1 -> Add2/1
  Gain6/1 -> Add2/2
  Add2/1 -> Product/1
  Gain4/1 -> Product/2
  Product1/1 -> Gain3/1
  Trigonometric Function1/1 -> Product1/2
  Ramp2/1 -> Gain7/1
  Gain7/1 -> Add1/1
  Ramp3/1 -> Gain8/1
  Gain8/1 -> Add1/2
  Add1/1 -> Product/3
  Constant/1 -> Add1/3
  Ramp6/1 -> Gain11/1
  Add3/1 -> Product1/3
  Constant1/1 -> Add3/3
  Gain12/1 -> Add3/2
  Gain9/1 -> Add4/1
  Add4/1 -> Product1/1
  Gain11/1 -> Add3/1
  Ramp4/1 -> Gain9/1
  Ramp7/1 -> Gain12/1
  Gain10/1 -> Add4/2
  Ramp5/1 -> Gain10/1

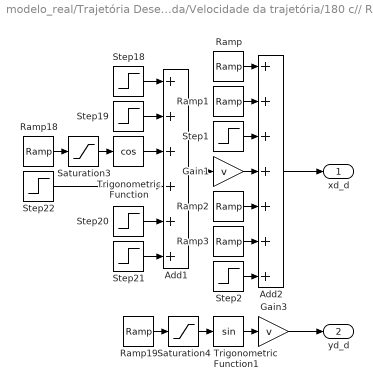
== system modelo_real/Trajetória Desejada/Velocidade da trajetória/180 c// RAMPA ==
  Add1 : Sum  Inputs=++++++
  Add2 : Sum  Inputs=+++++++
  Gain1 : Gain  Gain=v
  Gain3 : Gain  Gain=v
  Ramp : simulink/Sources/Ramp  slope=a  start=t_i  InitialOutput=0
  Ramp1 : simulink/Sources/Ramp  slope=-a  start=t_i_1  InitialOutput=0
  Ramp18 : simulink/Sources/Ramp  slope=pi/dur_c  start=t_i_c  InitialOutput=0
  Ramp19 : simulink/Sources/Ramp  slope=pi/dur_c  start=t_i_c  InitialOutput=0
  Ramp2 : simulink/Sources/Ramp  slope=a  start=t_i_3  InitialOutput=0
  Ramp3 : simulink/Sources/Ramp  slope=-a  start=t_f  InitialOutput=0
  Saturation3 : Saturate  UpperLimit=pi  LowerLimit=0
  Saturation4 : Saturate  UpperLimit=pi  LowerLimit=0
  Step1 : Step  Time=t_i_1  After=-v  SampleTime=0
  Step18 : Step  Time=t_i_1  SampleTime=0
  Step19 : Step  Time=t_i_c  After=-1  SampleTime=0
  Step2 : Step  Time=t_i_3  After=-v  SampleTime=0
  Step20 : Step  Time=t_i_3  SampleTime=0
  Step21 : Step  Time=t_f  After=-1  SampleTime=0
  Step22 : Step  Time=t_i_c  Before=-1  After=0  SampleTime=0
  Trigonometric Function : Trigonometry  Operator=cos
  Trigonometric Function1 : Trigonometry
  xd_d : Outport
  yd_d : Outport  Port=2
  wires:
  Add1/1 -> Gain1/1
  Ramp18/1 -> Saturation3/1
  Saturation3/1 -> Trigonometric Function/1
  Saturation4/1 -> Trigonometric Function1/1
  Ramp19/1 -> Saturation4/1
  Step18/1 -> Add1/1
  Step19/1 -> Add1/2
  Trigonometric Function/1 -> Add1/3
  Step22/1 -> Add1/4
  Add2/1 -> xd_d/1
  Ramp/1 -> Add2/1
  Ramp1/1 -> Add2/2
  Step1/1 -> Add2/3
  Gain1/1 -> Add2/4
  Gain3/1 -> yd_d/1
  Ramp2/1 -> Add2/5
  Ramp3/1 -> Add2/6
  Step20/1 -> Add1/5
  Step21/1 -> Add1/6
  Step2/1 -> Add2/7
  Trigonometric Function1/1 -> Gain3/1

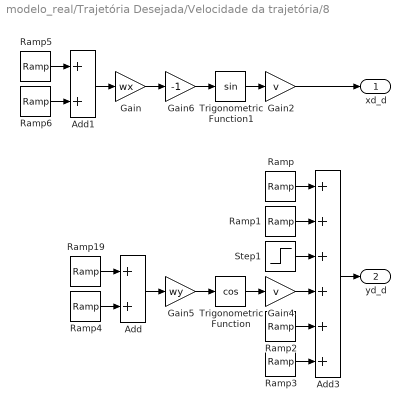
== system modelo_real/Trajetória Desejada/Velocidade da trajetória/8 ==
  Add : Sum
  Add1 : Sum
  Add3 : Sum  Inputs=++++++
  Gain : Gain  Gain=wx
  Gain2 : Gain  Gain=v
  Gain4 : Gain  Gain=v
  Gain5 : Gain  Gain=wy
  Gain6 : Gain  Gain=-1
  Ramp : simulink/Sources/Ramp  slope=a  start=t_i  InitialOutput=0
  Ramp1 : simulink/Sources/Ramp  slope=-a  start=t_i_1  InitialOutput=0
  Ramp19 : simulink/Sources/Ramp  slope=1  start=t_i_1  InitialOutput=0
  Ramp2 : simulink/Sources/Ramp  slope=-a  start=t_i_2  InitialOutput=0
  Ramp3 : simulink/Sources/Ramp  slope=a  start=t_f  InitialOutput=0
  Ramp4 : simulink/Sources/Ramp  slope=-1  start=t_i_2  InitialOutput=0
  Ramp5 : simulink/Sources/Ramp  slope=1  start=t_i_1  InitialOutput=0
  Ramp6 : simulink/Sources/Ramp  slope=-1  start=t_i_2  InitialOutput=0
  Step1 : Step  Time=t_i  After=-v  SampleTime=0
  Trigonometric Function : Trigonometry  Operator=cos
  Trigonometric Function1 : Trigonometry
  xd_d : Outport
  yd_d : Outport  Port=2
  wires:
  Add1/1 -> Gain/1
  Trigonometric Function/1 -> Gain4/1
  Trigonometric Function1/1 -> Gain2/1
  Add3/1 -> yd_d/1
  Gain/1 -> Gain6/1
  Gain5/1 -> Trigonometric Function/1
  Gain6/1 -> Trigonometric Function1/1
  Gain4/1 -> Add3/4
  Ramp2/1 -> Add3/5
  Ramp3/1 -> Add3/6
  Ramp1/1 -> Add3/2
  Ramp/1 -> Add3/1
  Step1/1 -> Add3/3
  Ramp19/1 -> Add/1
  Add/1 -> Gain5/1
  Ramp4/1 -> Add/2
  Ramp6/1 -> Add1/2
  Ramp5/1 -> Add1/1
  Gain2/1 -> xd_d/1

== system modelo_real/Trajetória Desejada/Velocidade da trajetória/90  ==
  Add7 : Sum  Inputs=++++
  Add8 : Sum  Inputs=++++
  Gain1 : Gain  Gain=v
  Gain3 : Gain  Gain=v
  Ramp18 : simulink/Sources/Ramp  slope=(pi/2)/time_c  start=t_i_c  InitialOutput=0
  Ramp19 : simulink/Sources/Ramp  slope=(pi/2)/time_c  start=t_i_c  InitialOutput=0
  Saturation3 : Saturate  UpperLimit=pi/2  LowerLimit=0
  Saturation4 : Saturate  UpperLimit=pi/2  LowerLimit=0
  Step18 : Step  Time=t_i  SampleTime=0
  Step19 : Step  Time=t_i_c  After=-1  SampleTime=0
  Step20 : Step  Time=t_i_2  SampleTime=0
  Step21 : Step  Time=t_f  After=-1  SampleTime=0
  Step22 : Step  Time=t_i_c  Before=-1  After=0  SampleTime=0
  Step23 : Step  Time=t_i_2  After=-1  SampleTime=0
  Trigonometric Function : Trigonometry  Operator=cos
  Trigonometric Function1 : Trigonometry
  xd_d : Outport
  yd_d : Outport  Port=2
  wires:
  Add7/1 -> Gain1/1
  Ramp18/1 -> Saturation3/1
  Step21/1 -> Add8/4
  Saturation3/1 -> Trigonometric Function/1
  Add8/1 -> Gain3/1
  Step20/1 -> Add8/3
  Trigonometric Function1/1 -> Add8/1
  Saturation4/1 -> Trigonometric Function1/1
  Ramp19/1 -> Saturation4/1
  Step23/1 -> Add8/2
  Gain1/1 -> xd_d/1
  Gain3/1 -> yd_d/1
  Step22/1 -> Add7/4
  Trigonometric Function/1 -> Add7/3
  Step19/1 -> Add7/2
  Step18/1 -> Add7/1

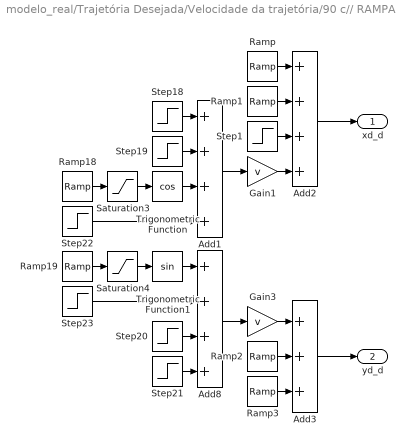
== system modelo_real/Trajetória Desejada/Velocidade da trajetória/90 c// RAMPA ==
  Add1 : Sum  Inputs=++++
  Add2 : Sum  Inputs=++++
  Add3 : Sum  Inputs=+++
  Add8 : Sum  Inputs=++++
  Gain1 : Gain  Gain=v
  Gain3 : Gain  Gain=v
  Ramp : simulink/Sources/Ramp  slope=a  start=t_i  InitialOutput=0
  Ramp1 : simulink/Sources/Ramp  slope=-a  start=t_i_1  InitialOutput=0
  Ramp18 : simulink/Sources/Ramp  slope=(pi/2)/dur_c  start=t_i_c  InitialOutput=0
  Ramp19 : simulink/Sources/Ramp  slope=(pi/2)/dur_c  start=t_i_c  InitialOutput=0
  Ramp2 : simulink/Sources/Ramp  slope=-a  start=t_i_3  InitialOutput=0
  Ramp3 : simulink/Sources/Ramp  slope=a  start=t_f  InitialOutput=0
  Saturation3 : Saturate  UpperLimit=pi/2  LowerLimit=0
  Saturation4 : Saturate  UpperLimit=pi/2  LowerLimit=0
  Step1 : Step  Time=t_i_1  After=-v  SampleTime=0
  Step18 : Step  Time=t_i_1  SampleTime=0
  Step19 : Step  Time=t_i_c  After=-1  SampleTime=0
  Step20 : Step  Time=t_i_2  SampleTime=0
  Step21 : Step  Time=t_f  After=-1  SampleTime=0
  Step22 : Step  Time=t_i_c  Before=-1  After=0  SampleTime=0
  Step23 : Step  Time=t_i_2  After=-1  SampleTime=0
  Trigonometric Function : Trigonometry  Operator=cos
  Trigonometric Function1 : Trigonometry
  xd_d : Outport
  yd_d : Outport  Port=2
  wires:
  Add1/1 -> Gain1/1
  Ramp18/1 -> Saturation3/1
  Step21/1 -> Add8/4
  Saturation3/1 -> Trigonometric Function/1
  Add8/1 -> Gain3/1
  Step20/1 -> Add8/3
  Trigonometric Function1/1 -> Add8/1
  Saturation4/1 -> Trigonometric Function1/1
  Ramp19/1 -> Saturation4/1
  Step23/1 -> Add8/2
  Step18/1 -> Add1/1
  Step19/1 -> Add1/2
  Trigonometric Function/1 -> Add1/3
  Step22/1 -> Add1/4
  Add2/1 -> xd_d/1
  Ramp/1 -> Add2/1
  Ramp1/1 -> Add2/2
  Step1/1 -> Add2/3
  Gain1/1 -> Add2/4
  Gain3/1 -> Add3/1
  Add3/1 -> yd_d/1
  Ramp2/1 -> Add3/2
  Ramp3/1 -> Add3/3

== system modelo_real/Trajetória Desejada/Velocidade da trajetória/Reta c// RAMPA ==
  Add1 : Sum
  Add2 : Sum  Inputs=++++++
  Constant : Constant  Value=0
  Gain1 : Gain  Gain=v
  Ramp : simulink/Sources/Ramp  slope=a  start=t_i  InitialOutput=0
  Ramp1 : simulink/Sources/Ramp  slope=-a  start=t_i_1  InitialOutput=0
  Ramp2 : simulink/Sources/Ramp  slope=-a  start=t_i_2  InitialOutput=0
  Step1 : Step  Time=t_i_1  After=-v  SampleTime=0
  Step18 : Step  Time=t_i_1  SampleTime=0
  Step19 : Step  Time=t_i_2  After=-1  SampleTime=0
  Step2 : Step  Time=t_i_2  After=v  SampleTime=0
  xd_d : Outport
  yd_d : Outport  Port=2
  wires:
  Add1/1 -> Gain1/1
  Step18/1 -> Add1/1
  Step19/1 -> Add1/2
  Add2/1 -> xd_d/1
  Ramp/1 -> Add2/1
  Ramp1/1 -> Add2/2
  Step1/1 -> Add2/3
  Gain1/1 -> Add2/4
  Ramp2/1 -> Add2/5
  Step2/1 -> Add2/6
  Constant/1 -> yd_d/1

== matlab function modelo_real/Modelo Real/Obtenção dos estados/Obtensão dos Estados ==
  data: cte input; thetaD input; thetaD_d input; thetaE input; thetaE_d input; xr_d output; yr_d output; phi output; x0_3 input
function [xr_d, yr_d, phi] = fcn(cte, thetaD, thetaD_d, thetaE, thetaE_d, x0_3)
%#codegen
% Parametros de simulação--------------------------------------------------
b   = cte(1,1);
c_d = cte(1,2);
c_e = cte(1,3);
L   = cte(1,4);

phi = c_d*thetaD - c_e*thetaE + x0_3;

% Cálculo de D e u---------------------------------------------------------
J = [c_d*b*cos(phi)-L*c_d*sin(phi), c_e*b*cos(phi)+L*c_e*sin(phi);
     c_d*b*sin(phi)+L*c_d*cos(phi), c_e*b*sin(phi)-L*c_e*cos(phi);
                               c_d,                          -c_e];
eta = [thetaD_d;
       thetaE_d];
 
% Cálculo de x_d-----------------------------------------------------------
x_d = J*eta;
xr_d  = x_d(1,1);
yr_d  = x_d(2,1);

== matlab function modelo_real/Equação Linearizante/Modelo do WMR ==
  data: cte input; u input; x input; thetaD_d output; thetaE_d output
function [thetaD_d, thetaE_d] = fcn(cte, u, x)
%#codegen
% Parametros de simulação--------------------------------------------------
b   = cte(1,1);
c_d = cte(1,2);
c_e = cte(1,3);
L   = cte(1,4);

phi = x(3,1);

% Cálculo de D e u---------------------------------------------------------
D = [c_d*b*cos(phi)-c_d*L*sin(phi) c_e*b*cos(phi)+c_e*L*sin(phi);
     c_d*b*sin(phi)+c_d*L*cos(phi) c_e*b*sin(phi)-c_e*L*cos(phi)];

eta = D^-1*(u);
 
% Cálculo de x_d-----------------------------------------------------------
thetaD_d = eta(1,1);
thetaE_d = eta(2,1);

== matlab function modelo_real/Modelo Real/Filtro D/Média ==
  data: u input; y output
function y = fcn(u)
y = mean(u);

== matlab function modelo_real/Modelo Real/Filtro E/Média ==
  data: u input; y output
function y = fcn(u)
y = mean(u);

== matlab function modelo_real/Estados/Estados ==
  data: xr output; yr output; x input; phi output
function [xr, yr, phi] = fcn(x)

%#codegen
%--------------------------------------------------------------------------
xr  = x(1,1);
yr  = x(2,1);
phi = x(3,1);

== matlab function modelo_real/Saída/Saídas ==
  data: xr output; yr output; x input
function [xr, yr] = fcn(x)

%#codegen
xr     = x(1,1);
yr     = x(2,1);
